simulink model "ZSM_TeslaModelS_statKreisfahrt"  (R2020b)
settings: Solver=FixedStepDiscrete  StartTime=0.0  StopTime=simtime  FixedStep=stepsize  RelTol=1e-3
undefined symbols (not defined in the file): activate_stop, activate_stop_vmax, ay_stop, ayObs, ayStiff, Bat_param, deltav_ist, DiscIntNeverNeededParam, EG_wunsch, magnitude, mu_road_LF, mu_road_LR, mu_road_RF, mu_road_RR, par_ASR, par_MDT, par_TIR, par_VEH, select_delta_h, select_M_wheel, stepsize, t, temp_betriebsstrategie, temperature_LTrange, track_left, track_right
libraries: Library_ASK x36, simulink x16, pid_lib x2, dspstat3 x2, Library_Betriebsstrategie x2, vehicle_model x2, pacejka_trans x1
(part 6 of 7)

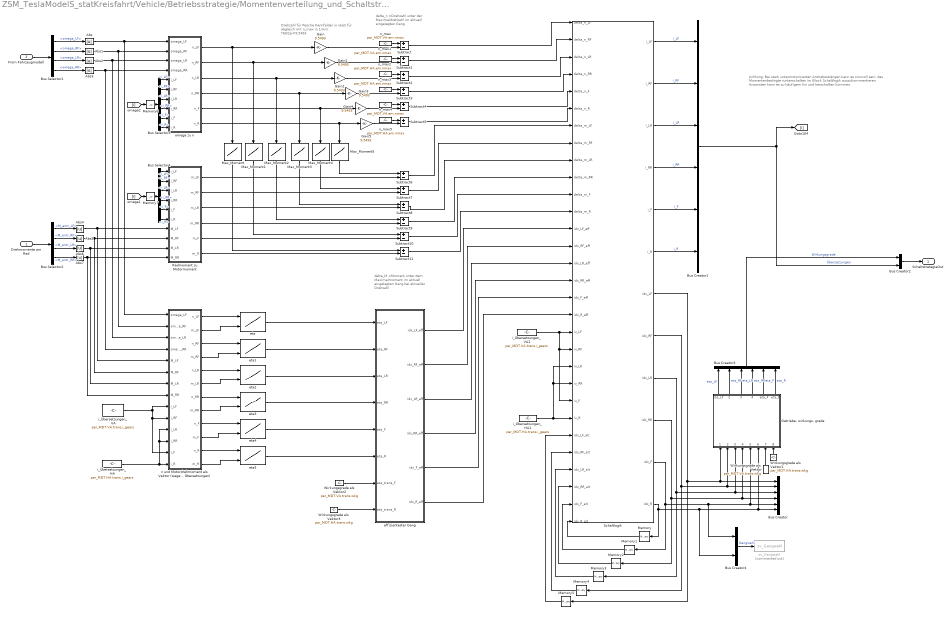
== system ZSM_TeslaModelS_statKreisfahrt/Vehicle/Betriebsstrategie/Momentenverteilung_und_Schaltstrategie1/Radmomentenaufteilung (Standardfahrmanöver)/Schaltstrategie ==
  note: Drehzahl für Pesche Kennfelder in rad/s
      | für abgleich mit n_max in 1/min
      | *60/2pi=9.5493
  note: Achtung: Bei stark untermotorisierten Antriebssträngen kann es sinnvoll sein,
      | das Momentenbedingte runterschalten im Block Schaltlogik auszukommentieren.
      | Ansonsten kann es zu häufigem hin und herschalten kommen.
  note: delta_M =Moment unter dem Maximalmoment im aktuell eingelegten Gang bei aktueller Drehzahl
  note: delta_n =Drehzahl unter der Maximaldrehzahl im aktuell eingelegten Gang
  Drehmomente am Rad : Inport
  From Fahrzeugmodell : Inport  Port=2
  Abs{,1..7} (8 alike) : Abs
  Bus Creator : BusCreator  Inputs=6
  Bus Creator1 : BusCreator  Inputs=6
  Bus Creator2 : BusCreator  Inputs=2
  Bus Creator3 : BusCreator  Inputs=6
  Bus Creator4 : BusCreator  Inputs=2
  Bus Selector1 : BusSelector  OutputSignals=omega.omega_LF,omega.omega_RF,omega.omega_LR,omega.omega_RR
  Bus Selector2 : BusSelector  OutputSignals=M_antr_LF,M_antr_RF,M_antr_LR,M_antr_RR
  Bus Selector3 : BusSelector  OutputSignals=i_LF,i_RF,i_LR,i_RR,i_F,i_R
  Bus Selector4 : BusSelector  OutputSignals=i_LF,i_RF,i_LR,i_RR,i_F,i_R
  Gain{,1..5} (6 alike) : Gain  Gain=9.5493
  Getriebe- wirkungs- grade : MATLAB Function  TreatAsAtomicUnit=on
  Max_Moment : Lookup_n-D  NumberOfTableDimensions=1  BreakpointsForDimension1=par_MDT.VA.em.MaxMotorTrqCurve_w  Table=par_MDT.VA.em.MaxMotorTrqCurve_M  InternalRulePriority=Speed  RndMeth=Simplest  InputSameDT=on
  Max_Moment1 : Lookup_n-D  NumberOfTableDimensions=1  BreakpointsForDimension1=par_MDT.VA.em.MaxMotorTrqCurve_w  Table=par_MDT.VA.em.MaxMotorTrqCurve_M  InternalRulePriority=Speed  RndMeth=Simplest  InputSameDT=on
  Max_Moment2 : Lookup_n-D  NumberOfTableDimensions=1  BreakpointsForDimension1=par_MDT.HA.em.MaxMotorTrqCurve_w  Table=par_MDT.HA.em.MaxMotorTrqCurve_M  InternalRulePriority=Speed  RndMeth=Simplest  InputSameDT=on
  Max_Moment3 : Lookup_n-D  NumberOfTableDimensions=1  BreakpointsForDimension1=par_MDT.HA.em.MaxMotorTrqCurve_w  Table=par_MDT.HA.em.MaxMotorTrqCurve_M  InternalRulePriority=Speed  RndMeth=Simplest  InputSameDT=on
  Max_Moment4 : Lookup_n-D  NumberOfTableDimensions=1  BreakpointsForDimension1=par_MDT.VA.em.MaxMotorTrqCurve_w  Table=par_MDT.VA.em.MaxMotorTrqCurve_M  InternalRulePriority=Speed  RndMeth=Simplest  InputSameDT=on
  Max_Moment5 : Lookup_n-D  NumberOfTableDimensions=1  BreakpointsForDimension1=par_MDT.HA.em.MaxMotorTrqCurve_w  Table=par_MDT.HA.em.MaxMotorTrqCurve_M  InternalRulePriority=Speed  RndMeth=Simplest  InputSameDT=on
  Memory{,1..7} (8 alike) : Memory  InitialCondition=1
  Radmoment zu Motormoment : MATLAB Function  TreatAsAtomicUnit=on
  Schaltlogik : MATLAB Function  TreatAsAtomicUnit=on
  Subtract{,1..11} (12 alike) : Sum  Inputs=+-
  Wirkungsgrade als Vektor : Constant  Value=par_MDT.VA.trans.wkg
  Wirkungsgrade als Vektor1 : Constant  Value=par_MDT.HA.trans.wkg
  Wirkungsgrade als Vektor2 : Constant  Value=par_MDT.VA.trans.wkg
  Wirkungsgrade als Vektor3 : Constant  Value=par_MDT.HA.trans.wkg
  effizientester Gang : MATLAB Function  TreatAsAtomicUnit=on
  eta : Lookup_n-D  BreakpointsForDimension1=par_MDT.VA.em.MotorEffMap3D_w  BreakpointsForDimension2=par_MDT.VA.em.MotorEffMap3D_M  Table=par_MDT.VA.em.MotorEffMap3D  InternalRulePriority=Speed  RndMeth=Simplest  InputSameDT=on
      settings: InputPortMap=u0,u1
  eta1 : Lookup_n-D  BreakpointsForDimension1=par_MDT.VA.em.MotorEffMap3D_w  BreakpointsForDimension2=par_MDT.VA.em.MotorEffMap3D_M  Table=par_MDT.VA.em.MotorEffMap3D  InternalRulePriority=Speed  RndMeth=Simplest  InputSameDT=on
      settings: InputPortMap=u0,u1
  eta2 : Lookup_n-D  BreakpointsForDimension1=par_MDT.HA.em.MotorEffMap3D_w  BreakpointsForDimension2=par_MDT.HA.em.MotorEffMap3D_M  Table=par_MDT.HA.em.MotorEffMap3D  InternalRulePriority=Speed  RndMeth=Simplest  InputSameDT=on
      settings: InputPortMap=u0,u1
  eta3 : Lookup_n-D  BreakpointsForDimension1=par_MDT.HA.em.MotorEffMap3D_w  BreakpointsForDimension2=par_MDT.HA.em.MotorEffMap3D_M  Table=par_MDT.HA.em.MotorEffMap3D  InternalRulePriority=Speed  RndMeth=Simplest  InputSameDT=on
      settings: InputPortMap=u0,u1
  eta4 : Lookup_n-D  BreakpointsForDimension1=par_MDT.VA.em.MotorEffMap3D_w  BreakpointsForDimension2=par_MDT.VA.em.MotorEffMap3D_M  Table=par_MDT.VA.em.MotorEffMap3D  InternalRulePriority=Speed  RndMeth=Simplest  InputSameDT=on
      settings: InputPortMap=u0,u1
  eta5 : Lookup_n-D  BreakpointsForDimension1=par_MDT.HA.em.MotorEffMap3D_w  BreakpointsForDimension2=par_MDT.HA.em.MotorEffMap3D_M  Table=par_MDT.HA.em.MotorEffMap3D  InternalRulePriority=Speed  RndMeth=Simplest  InputSameDT=on
      settings: InputPortMap=u0,u1
  i_Übersetzungen_HA : Constant  Value=par_MDT.HA.trans.i_gears
  i_Übersetzungen_HA1 : Constant  Value=par_MDT.HA.trans.i_gears
  i_Übersetzungen_VA : Constant  Value=par_MDT.VA.trans.i_gears
  i_Übersetzungen_VA1 : Constant  Value=par_MDT.VA.trans.i_gears
  n und Motordrehmoment als Vektor (wegen ALLEN Übersetzungen) : MATLAB Function  TreatAsAtomicUnit=on
  n_max : Constant  Value=par_MDT.VA.em.nmax
  n_max1 : Constant  Value=par_MDT.VA.em.nmax
  n_max2 : Constant  Value=par_MDT.HA.em.nmax
  n_max3 : Constant  Value=par_MDT.HA.em.nmax
  n_max4 : Constant  Value=par_MDT.VA.em.nmax
  n_max5 : Constant  Value=par_MDT.HA.em.nmax
  omega zu n : MATLAB Function  TreatAsAtomicUnit=on
  sv_Gangwahl : ToWorkspace  Commented=on  VariableName=sv_Gangwahl  SaveFormat=Timeseries  SampleTime=-1
      settings: Decimation=savedec
  SchaltstrategieOut : Outport  VectorParamsAs1DForOutWhenUnconnected=off
  wires:
  Abs7/1 -> n und Motordrehmoment als Vektor (wegen ALLEN Übersetzungen)/8(M_RR), Radmoment zu Motormoment/10(M_RR)
  Abs6/1 -> n und Motordrehmoment als Vektor (wegen ALLEN Übersetzungen)/7(M_LR), Radmoment zu Motormoment/9(M_LR)
  Abs5/1 -> n und Motordrehmoment als Vektor (wegen ALLEN Übersetzungen)/6(M_RF), Radmoment zu Motormoment/8(M_RF)
  Abs4/1 -> n und Motordrehmoment als Vektor (wegen ALLEN Übersetzungen)/5(M_LF), Radmoment zu Motormoment/7(M_LF)
  Abs3/1 -> n und Motordrehmoment als Vektor (wegen ALLEN Übersetzungen)/4(omega_RR), omega zu n/4(omega_RR)
  Abs2/1 -> n und Motordrehmoment als Vektor (wegen ALLEN Übersetzungen)/3(omega_LR), omega zu n/3(omega_LR)
  Abs1/1 -> n und Motordrehmoment als Vektor (wegen ALLEN Übersetzungen)/2(omega_RF), omega zu n/2(omega_RF)
  Abs/1 -> n und Motordrehmoment als Vektor (wegen ALLEN Übersetzungen)/1(omega_LF), omega zu n/1(omega_LF)
  omega zu n/6(n_R) -> Gain5/1, Max_Moment5/1
  omega zu n/1(n_LF) -> Gain/1, Max_Moment/1
  omega zu n/5(n_F) -> Max_Moment4/1, Gain4/1
  omega zu n/4(n_RR) -> Max_Moment3/1, Gain3/1
  omega zu n/3(n_LR) -> Max_Moment2/1, Gain2/1
  omega zu n/2(n_RF) -> Max_Moment1/1, Gain1/1
  Bus Selector1/4 -> Abs3/1  "<omega_RR>"
  Bus Selector1/3 -> Abs2/1  "<omega_LR>"
  Bus Selector1/2 -> Abs1/1  "<omega_RF>"
  Bus Selector1/1 -> Abs/1  "<omega_LF>"
  Drehmomente am Rad/1 -> Bus Selector2/1
  From Fahrzeugmodell/1 -> Bus Selector1/1
  Bus Selector2/1 -> Abs4/1  "<M_antr_LF>"
  Bus Selector2/2 -> Abs5/1  "<M_antr_RF>"
  Bus Selector2/3 -> Abs6/1  "<M_antr_LR>"
  Bus Selector2/4 -> Abs7/1  "<M_antr_RR>"
  n_max/1 -> Subtract/1
  n_max1/1 -> Subtract1/1
  n_max2/1 -> Subtract2/1
  n_max3/1 -> Subtract3/1
  n_max4/1 -> Subtract4/1
  n_max5/1 -> Subtract5/1
  Radmoment zu Motormoment/1(m_LF) -> Subtract6/2
  Radmoment zu Motormoment/2(m_RF) -> Subtract7/2
  Radmoment zu Motormoment/3(m_LR) -> Subtract8/2
  Radmoment zu Motormoment/4(m_RR) -> Subtract9/2
  Radmoment zu Motormoment/5(m_F) -> Subtract10/2
  Radmoment zu Motormoment/6(m_R) -> Subtract11/2
  Max_Moment5/1 -> Subtract6/1
  Max_Moment4/1 -> Subtract7/1
  Max_Moment3/1 -> Subtract8/1
  Max_Moment2/1 -> Subtract9/1
  Max_Moment1/1 -> Subtract10/1
  Max_Moment/1 -> Subtract11/1
  i_Übersetzungen_VA/1 -> n und Motordrehmoment als Vektor (wegen ALLEN Übersetzungen)/9(i_LF), n und Motordrehmoment als Vektor (wegen ALLEN Übersetzungen)/13(i_F), n und Motordrehmoment als Vektor (wegen ALLEN Übersetzungen)/10(i_RF)
  n und Motordrehmoment als Vektor (wegen ALLEN Übersetzungen)/1(n_LF) -> eta/1
  n und Motordrehmoment als Vektor (wegen ALLEN Übersetzungen)/2(m_LF) -> eta/2
  n und Motordrehmoment als Vektor (wegen ALLEN Übersetzungen)/3(n_RF) -> eta1/1
  n und Motordrehmoment als Vektor (wegen ALLEN Übersetzungen)/4(m_RF) -> eta1/2
  n und Motordrehmoment als Vektor (wegen ALLEN Übersetzungen)/5(n_LR) -> eta2/1
  n und Motordrehmoment als Vektor (wegen ALLEN Übersetzungen)/6(m_LR) -> eta2/2
  n und Motordrehmoment als Vektor (wegen ALLEN Übersetzungen)/7(n_RR) -> eta3/1
  n und Motordrehmoment als Vektor (wegen ALLEN Übersetzungen)/8(m_RR) -> eta3/2
  n und Motordrehmoment als Vektor (wegen ALLEN Übersetzungen)/9(n_F) -> eta4/1
  n und Motordrehmoment als Vektor (wegen ALLEN Übersetzungen)/10(m_F) -> eta4/2
  n und Motordrehmoment als Vektor (wegen ALLEN Übersetzungen)/11(n_R) -> eta5/1
  n und Motordrehmoment als Vektor (wegen ALLEN Übersetzungen)/12(m_R) -> eta5/2
  eta/1 -> effizientester Gang/1(eta_LF)
  eta1/1 -> effizientester Gang/2(eta_RF)
  eta2/1 -> effizientester Gang/3(eta_LR)
  eta3/1 -> effizientester Gang/4(eta_RR)
  eta4/1 -> effizientester Gang/5(eta_F)
  eta5/1 -> effizientester Gang/6(eta_R)
  Subtract/1 -> Schaltlogik/1(delta_n_LF)
  Subtract1/1 -> Schaltlogik/2(delta_n_RF)
  Subtract2/1 -> Schaltlogik/3(delta_n_LR)
  Subtract3/1 -> Schaltlogik/4(delta_n_RR)
  Subtract4/1 -> Schaltlogik/5(delta_n_F)
  Subtract5/1 -> Schaltlogik/6(delta_n_R)
  Subtract6/1 -> Schaltlogik/7(delta_m_LF)
  Subtract7/1 -> Schaltlogik/8(delta_m_RF)
  Subtract8/1 -> Schaltlogik/9(delta_m_LR)
  Subtract9/1 -> Schaltlogik/10(delta_m_RR)
  Subtract10/1 -> Schaltlogik/11(delta_m_F)
  Subtract11/1 -> Schaltlogik/12(delta_m_R)
  effizientester Gang/1(idx_LF_eff) -> Schaltlogik/13(idx_LF_eff)
  effizientester Gang/2(idx_RF_eff) -> Schaltlogik/14(idx_RF_eff)
  effizientester Gang/3(idx_LR_eff) -> Schaltlogik/15(idx_LR_eff)
  effizientester Gang/4(idx_RR_eff) -> Schaltlogik/16(idx_RR_eff)
  effizientester Gang/5(idx_F_eff) -> Schaltlogik/17(idx_F_eff)
  effizientester Gang/6(idx_R_eff) -> Schaltlogik/18(idx_R_eff)
  Schaltlogik/12(idx_R) -> Memory/1, Bus Creator4/2, Getriebe- wirkungs- grade/6(idx_R), Bus Creator/6
  Schaltlogik/11(idx_F) -> Memory1/1, Bus Creator4/1, Bus Creator/5, Getriebe- wirkungs- grade/5(idx_F)
  Schaltlogik/9(idx_LR) -> Memory3/1, Bus Creator/3, Getriebe- wirkungs- grade/3(idx_LR)
  Schaltlogik/8(idx_RF) -> Memory4/1, Bus Creator/2, Getriebe- wirkungs- grade/2(idx_RF)
  Schaltlogik/7(idx_LF) -> Memory5/1, Bus Creator/1, Getriebe- wirkungs- grade/1(idx_LF)
  Memory/1 -> Schaltlogik/30(idx_R_alt)
  Memory1/1 -> Schaltlogik/29(idx_F_alt)
  Memory2/1 -> Schaltlogik/28(idx_RR_alt)
  Memory3/1 -> Schaltlogik/27(idx_LR_alt)
  Memory4/1 -> Schaltlogik/26(idx_RF_alt)
  Memory5/1 -> Schaltlogik/25(idx_LF_alt)
  Schaltlogik/10(idx_RR) -> Memory2/1, Bus Creator/4, Getriebe- wirkungs- grade/4(idx_RR)
  Schaltlogik/1(i_LF) -> Bus Creator1/1  "i_LF"
  Schaltlogik/2(i_RF) -> Bus Creator1/2  "i_RF"
  Schaltlogik/3(i_LR) -> Bus Creator1/3  "i_LR"
  Schaltlogik/4(i_RR) -> Bus Creator1/4  "i_RR"
  Schaltlogik/5(i_F) -> Bus Creator1/5  "i_F"
  Schaltlogik/6(i_R) -> Bus Creator1/6  "i_R"
  Bus Selector3/1 -> omega zu n/5(i_LF)  "<i_LF>"
  [i] -> Memory6/1
  Bus Selector3/2 -> omega zu n/6(i_RF)  "<i_RF>"
  Bus Selector3/3 -> omega zu n/7(i_LR)  "<i_LR>"
  Bus Selector3/4 -> omega zu n/8(i_RR)  "<i_RR>"
  Bus Selector3/5 -> omega zu n/9(i_F)  "<i_F>"
  Bus Selector3/6 -> omega zu n/10(i_R)  "<i_R>"
  Memory6/1 -> Bus Selector3/1
  [i] -> Memory7/1
  Memory7/1 -> Bus Selector4/1
  Bus Selector4/1 -> Radmoment zu Motormoment/1(i_LF)  "<i_LF>"
  Bus Selector4/2 -> Radmoment zu Motormoment/2(i_RF)  "<i_RF>"
  Bus Selector4/3 -> Radmoment zu Motormoment/3(i_LR)  "<i_LR>"
  Bus Selector4/4 -> Radmoment zu Motormoment/4(i_RR)  "<i_RR>"
  Bus Selector4/5 -> Radmoment zu Motormoment/5(i_F)  "<i_F>"
  Bus Selector4/6 -> Radmoment zu Motormoment/6(i_R)  "<i_R>"
  i_Übersetzungen_HA/1 -> n und Motordrehmoment als Vektor (wegen ALLEN Übersetzungen)/11(i_LR), n und Motordrehmoment als Vektor (wegen ALLEN Übersetzungen)/12(i_RR), n und Motordrehmoment als Vektor (wegen ALLEN Übersetzungen)/14(i_R)
  i_Übersetzungen_VA1/1 -> Schaltlogik/23(iv_F), Schaltlogik/20(iv_RF), Schaltlogik/19(iv_LF)
  i_Übersetzungen_HA1/1 -> Schaltlogik/21(iv_LR), Schaltlogik/22(iv_RR), Schaltlogik/24(iv_R)
  Gain/1 -> Subtract/2
  Gain1/1 -> Subtract1/2
  Gain2/1 -> Subtract2/2
  Gain3/1 -> Subtract3/2
  Gain4/1 -> Subtract4/2
  Gain5/1 -> Subtract5/2
  Bus Creator1/1 -> Bus Creator2/2, [i]  "Übersetzungen"
  Bus Creator2/1 -> SchaltstrategieOut/1
  Wirkungsgrade als Vektor/1 -> Getriebe- wirkungs- grade/7(ETA_F)
  Wirkungsgrade als Vektor1/1 -> Getriebe- wirkungs- grade/8(ETA_R)
  Getriebe- wirkungs- grade/2(eta_RF) -> Bus Creator3/2  "eta_RF"
  Getriebe- wirkungs- grade/3(eta_LR) -> Bus Creator3/3  "eta_LR"
  Getriebe- wirkungs- grade/4(eta_RR) -> Bus Creator3/4  "eta_RR"
  Getriebe- wirkungs- grade/5(eta_F) -> Bus Creator3/5  "eta_F"
  Getriebe- wirkungs- grade/6(eta_R) -> Bus Creator3/6  "eta_R"
  Getriebe- wirkungs- grade/1(eta_LF) -> Bus Creator3/1  "eta_LF"
  Bus Creator3/1 -> Bus Creator2/1  "Wirkungsgrade"
  Wirkungsgrade als Vektor2/1 -> effizientester Gang/7(eta_trans_F)
  Wirkungsgrade als Vektor3/1 -> effizientester Gang/8(eta_trans_R)
  Bus Creator4/1 -> sv_Gangwahl/1  "Gangwahl"

== system ZSM_TeslaModelS_statKreisfahrt/Vehicle/Betriebsstrategie/Momentenverteilung_und_Schaltstrategie1/adaptive Limiter/Enabled Subsystem ==
  In1 : Inport
  Enable : EnablePort
  Out1 : Outport  VectorParamsAs1DForOutWhenUnconnected=off
  wires:
  In1/1 -> Out1/1

== system ZSM_TeslaModelS_statKreisfahrt/Vehicle/Betriebsstrategie/Momentenverteilung_und_Schaltstrategie1/adaptive Limiter/Enabled Subsystem1 ==
  In1 : Inport
  Enable : EnablePort
  Discrete-Time Integrator : DiscreteIntegrator  InitialCondition=1  SampleTime=-1  ICPrevOutput=DiscIntNeverNeededParam  ICPrevScaledInput=DiscIntNeverNeededParam
  Out1 : Outport  VectorParamsAs1DForOutWhenUnconnected=off
  wires:
  Discrete-Time Integrator/1 -> Out1/1
  In1/1 -> Discrete-Time Integrator/1

== system ZSM_TeslaModelS_statKreisfahrt/Vehicle/Betriebsstrategie/Momentenverteilung_und_Schaltstrategie1/Radmomentenaufteilung (Effizienz)/Limits ermitteln/Axle activator ==
  Add4 : Sum
  Add6 : Sum
  Constant3 : Constant  Value=par_MDT.AUS.akt.az_VA
  Constant4 : Constant  Value=par_MDT.AUS.akt.az_HA
  Constant5 : Constant  Value=par_MDT.AUS.akt.rn_HA
  Constant6 : Constant  Value=par_MDT.AUS.akt.rn_VA
  VA : Outport  VectorParamsAs1DForOutWhenUnconnected=off
  HA : Outport  Port=2  VectorParamsAs1DForOutWhenUnconnected=off
  wires:
  Add4/1 -> VA/1
  Constant6/1 -> Add4/2
  Constant3/1 -> Add4/1
  Constant5/1 -> Add6/2
  Add6/1 -> HA/1
  Constant4/1 -> Add6/1

== system ZSM_TeslaModelS_statKreisfahrt/Vehicle/Betriebsstrategie/Momentenverteilung_und_Schaltstrategie1/Radmomentenaufteilung (Effizienz)/Limits ermitteln/Falls M_wheel kleiner als M_VA_pot ==
  M_VA_pot_in : Inport
  M_wheel : Inport  Port=2
  Rekuindex : Inport  Port=3
  M_HA_pot_in : Inport  Port=4
  Abs : Abs
  Abs1 : Abs
  Abs2 : Abs
  MinMax : MinMax  Inputs=2
  MinMax1 : MinMax  Inputs=2
  Product : Product
  Product1 : Product
  M_VA_pot_out : Outport  VectorParamsAs1DForOutWhenUnconnected=off
  M_wheel_out : Outport  Port=2  VectorParamsAs1DForOutWhenUnconnected=off
  M_HA_pot_out : Outport  Port=3  VectorParamsAs1DForOutWhenUnconnected=off
  wires:
  Abs1/1 -> MinMax1/1, MinMax/2
  MinMax/1 -> Product/1
  Abs/1 -> MinMax/1
  M_VA_pot_in/1 -> Abs/1
  M_wheel/1 -> M_wheel_out/1, Abs1/1
  Rekuindex/1 -> Product1/1, Product/2
  Product/1 -> M_VA_pot_out/1
  Abs2/1 -> MinMax1/2
  M_HA_pot_in/1 -> Abs2/1
  MinMax1/1 -> Product1/2
  Product1/1 -> M_HA_pot_out/1

== system ZSM_TeslaModelS_statKreisfahrt/Vehicle/Betriebsstrategie/Momentenverteilung_und_Schaltstrategie1/Radmomentenaufteilung (Effizienz)/Momentenrückführung und Motormomentberechnung/Getriebewirkungsgradberechnung Hinterachse ==
  Rekuindex : Inport
  M_HA_mot : Inport  Port=2
  Abs : Abs
  Constant1 : Constant  Value=par_VEH.dt.ecu.Wirkungsgrade_HA
  Constant2 : Constant  Commented=on  Value=par_MDT.HA.em.M_max_achse
  Divide : Product  Commented=on  Inputs=*/
  Divide1 : Product  Inputs=/*
  Falls radnahe Maschine an HA1 : Subsystem
  Falls radnahe Maschine an HA2 : Subsystem
  MATLAB Function1 : MATLAB Function  Commented=on  TreatAsAtomicUnit=on
  Product : Product
  Switch : Switch  Commented=on  Criteria=u2 > Threshold  Threshold=0.15
  WKG_GTR_HA : Outport  VectorParamsAs1DForOutWhenUnconnected=off
  wires:
  Constant2/1 -> Divide/2, MATLAB Function1/2(M_max)
  Constant1/1 -> Divide1/1
  M_HA_mot/1 -> Abs/1
  Product/1 -> Falls radnahe Maschine an HA2/1(M_HA)
  Falls radnahe Maschine an HA1/1(M_HA_mot) -> Divide1/2
  ? -> Switch/1, Divide/1, MATLAB Function1/1(M_out)
  Switch/1 -> ?
  Rekuindex/1 -> Product/2
  Abs/1 -> Falls radnahe Maschine an HA1/1(M_HA)
  MATLAB Function1/1(M_in) -> Switch/3
  Divide/1 -> Switch/2
  Falls radnahe Maschine an HA2/1(M_HA_mot) -> WKG_GTR_HA/1
  Divide1/1 -> Product/1

== system ZSM_TeslaModelS_statKreisfahrt/Vehicle/Betriebsstrategie/Momentenverteilung_und_Schaltstrategie1/Radmomentenaufteilung (Effizienz)/Momentenrückführung und Motormomentberechnung/Getriebewirkungsgradberechnung Vorderachse ==
  M_VA_mot : Inport
  Rekuindex : Inport  Port=2
  Abs : Abs
  Constant5 : Constant  Value=par_VEH.dt.ecu.Wirkungsgrade_VA
  Constant6 : Constant  Commented=on  Value=par_MDT.VA.em.M_max_achse
  Divide : Product  Commented=on  Inputs=*/
  Divide4 : Product  Inputs=/*
  Falls radnahe Maschine an VA : Subsystem
  Falls radnahe Maschine an VA1 : Subsystem
  MATLAB Function : MATLAB Function  Commented=on  TreatAsAtomicUnit=on
  Product : Product
  Switch : Switch  Commented=on  Criteria=u2 > Threshold  Threshold=0.15
  WKG_GTR_VA : Outport  VectorParamsAs1DForOutWhenUnconnected=off
  wires:
  Constant6/1 -> Divide/2, MATLAB Function/2(M_max)
  Constant5/1 -> Divide4/1
  M_VA_mot/1 -> Abs/1
  Product/1 -> Falls radnahe Maschine an VA1/1(M_VA)
  Falls radnahe Maschine an VA/1(M_VA_mot) -> Divide4/2
  ? -> Switch/1, Divide/1, MATLAB Function/1(M_out)
  Switch/1 -> ?
  Rekuindex/1 -> Product/2
  Abs/1 -> Falls radnahe Maschine an VA/1(M_VA)
  MATLAB Function/1(M_in) -> Switch/3
  Divide/1 -> Switch/2
  Falls radnahe Maschine an VA1/1(M_VA_mot) -> WKG_GTR_VA/1
  Divide4/1 -> Product/1

== system ZSM_TeslaModelS_statKreisfahrt/Vehicle/Betriebsstrategie/Momentenverteilung_und_Schaltstrategie1/Radmomentenaufteilung (Effizienz)/Momentenrückführung und Motormomentberechnung/Subsystem ==
  M_VA_pot : Inport
  M_VA_mot_in : Inport  Port=2
  Enable : EnablePort
  Abs : Abs
  Abs1 : Abs
  Bias : Bias  Bias=0.01
  Constant1 : Constant  Value=par_VEH.dt.ecu.Wirkungsgrade_VA
  Constant4 : Constant  Value=NaN
  Divide : Product  Inputs=/*
  Relational Operator : RelationalOperator  Operator=<  OutDataTypeStr=boolean  RndMeth=Nearest
  Switch : Switch  Criteria=u2 > Threshold
  M_VA_mot_out : Outport  VectorParamsAs1DForOutWhenUnconnected=off
  wires:
  Abs/1 -> Relational Operator/2
  Switch/1 -> M_VA_mot_out/1
  Constant1/1 -> Divide/1
  M_VA_pot/1 -> Divide/2
  Bias/1 -> Relational Operator/1
  Relational Operator/1 -> Switch/2
  Constant4/1 -> Switch/1
  Divide/1 -> Abs1/1
  Abs1/1 -> Bias/1
  M_VA_mot_in/1 -> Switch/3, Abs/1

== system ZSM_TeslaModelS_statKreisfahrt/Vehicle/Betriebsstrategie/Momentenverteilung_und_Schaltstrategie1/Radmomentenaufteilung (Effizienz)/Momentenrückführung und Motormomentberechnung/Subsystem1 ==
  M_HA_pot : Inport
  M_HA_mot_in : Inport  Port=2
  Enable : EnablePort
  Abs : Abs
  Abs1 : Abs
  Bias : Bias  Bias=0.01
  Constant1 : Constant  Value=par_VEH.dt.ecu.Wirkungsgrade_HA
  Constant4 : Constant  Value=NaN
  Divide : Product  Inputs=/*
  Relational Operator : RelationalOperator  Operator=<  OutDataTypeStr=boolean  RndMeth=Nearest
  Switch : Switch  Criteria=u2 > Threshold
  M_HA_mot_out : Outport  VectorParamsAs1DForOutWhenUnconnected=off
  wires:
  Abs1/1 -> Bias/1
  Abs/1 -> Relational Operator/2
  Switch/1 -> M_HA_mot_out/1
  Bias/1 -> Relational Operator/1
  M_HA_mot_in/1 -> Switch/3, Abs/1
  Constant4/1 -> Switch/1
  Relational Operator/1 -> Switch/2
  Divide/1 -> Abs1/1
  M_HA_pot/1 -> Divide/2
  Constant1/1 -> Divide/1

== system ZSM_TeslaModelS_statKreisfahrt/Vehicle/Betriebsstrategie/Momentenverteilung_und_Schaltstrategie1/Radmomentenaufteilung (Effizienz)/Optimierung und Schaltstrategie/Bereinigung ==
  M_VA_in : Inport
  M_HA_in : Inport  Port=2
  Constant : Constant  Value=0
  Constant1 : Constant  Value=0
  Relational Operator : RelationalOperator  Operator=isNaN  OutDataTypeStr=boolean  RndMeth=Nearest
  Relational Operator1 : RelationalOperator  Operator=isNaN  OutDataTypeStr=boolean  RndMeth=Nearest
  Switch : Switch  Criteria=u2 > Threshold
  Switch1 : Switch  Criteria=u2 > Threshold
  M_VA_out : Outport  VectorParamsAs1DForOutWhenUnconnected=off
  M_HA_out : Outport  Port=2  VectorParamsAs1DForOutWhenUnconnected=off
  wires:
  Switch1/1 -> M_HA_out/1
  M_VA_in/1 -> Relational Operator/1, Switch/3
  Constant/1 -> Switch/1
  Switch/1 -> M_VA_out/1
  Constant1/1 -> Switch1/1
  Relational Operator1/1 -> Switch1/2
  M_HA_in/1 -> Relational Operator1/1, Switch1/3
  Relational Operator/1 -> Switch/2

== system ZSM_TeslaModelS_statKreisfahrt/Vehicle/Betriebsstrategie/Momentenverteilung_und_Schaltstrategie1/Radmomentenaufteilung (Effizienz)/Torque shift damper/Axle activator ==
  Add4 : Sum
  Add6 : Sum
  Constant3 : Constant  Value=par_MDT.AUS.akt.az_VA
  Constant4 : Constant  Value=par_MDT.AUS.akt.az_HA
  Constant5 : Constant  Value=par_MDT.AUS.akt.rn_HA
  Constant6 : Constant  Value=par_MDT.AUS.akt.rn_VA
  VA : Outport  VectorParamsAs1DForOutWhenUnconnected=off
  HA : Outport  Port=2  VectorParamsAs1DForOutWhenUnconnected=off
  wires:
  Add4/1 -> VA/1
  Constant6/1 -> Add4/2
  Constant3/1 -> Add4/1
  Constant5/1 -> Add6/2
  Add6/1 -> HA/1
  Constant4/1 -> Add6/1

== system ZSM_TeslaModelS_statKreisfahrt/Vehicle/Betriebsstrategie/Momentenverteilung_und_Schaltstrategie1/Radmomentenaufteilung (Effizienz)/Torque shift damper/Optimierung_damped_AWD ==
  P_achs : Inport
  M_target : Inport  Port=2
  Enable : EnablePort
  Constant : Constant  Value=0.022
  Constant1 : Constant  Value=2
  Memory : Memory  InitialCondition=1
  Memory1 : Memory
  Memory2 : Memory  InitialCondition=1
  Minimierung : MATLAB Function  TreatAsAtomicUnit=on
  Product : Product
  Sign : Signum
  P_opt : Outport  VectorParamsAs1DForOutWhenUnconnected=off
  ind : Outport  Port=2  VectorParamsAs1DForOutWhenUnconnected=off
  wires:
  P_achs/1 -> Minimierung/1(P_achs)
  M_target/1 -> Product/1, Minimierung/4(M_target), Memory2/1
  Constant/1 -> Minimierung/2(difference)
  Memory2/1 -> Product/2
  Constant1/1 -> Minimierung/3(max_oscillation_sec)
  Minimierung/2(ind) -> ind/1, Memory/1
  Memory1/1 -> Minimierung/7(count_prev)
  Memory/1 -> Minimierung/6(ind_prev)
  Minimierung/3(count) -> Memory1/1
  Minimierung/1(P_opt) -> P_opt/1
  Product/1 -> Sign/1
  Sign/1 -> Minimierung/5(change)

== system ZSM_TeslaModelS_statKreisfahrt/Vehicle/Betriebsstrategie/Momentenverteilung_und_Schaltstrategie1/Radmomentenaufteilung (Effizienz)/Torque shift damper/Optimierung_eine_achs ==
  P_achs : Inport
  M_target : Inport  Port=2
  Akt_VA : Inport  Port=3
  Akt_HA : Inport  Port=4
  Enable : EnablePort
  Optimierung : MATLAB Function  TreatAsAtomicUnit=on
  "P_opt " : Outport  VectorParamsAs1DForOutWhenUnconnected=off
  "ind " : Outport  Port=2  VectorParamsAs1DForOutWhenUnconnected=off
  wires:
  Optimierung/1(P_opt) -> "P_opt "/1
  Optimierung/2(ind) -> "ind "/1
  M_target/1 -> Optimierung/2(M_target)
  P_achs/1 -> Optimierung/1(P_achs)
  Akt_VA/1 -> Optimierung/3(VA)
  Akt_HA/1 -> Optimierung/4(HA)

== system ZSM_TeslaModelS_statKreisfahrt/Vehicle/Betriebsstrategie/Momentenverteilung_und_Schaltstrategie1/Radmomentenaufteilung (Effizienz)/Momentenrückführung und Motormomentberechnung/Getriebewirkungsgradberechnung Hinterachse/Falls radnahe Maschine an HA1 ==
  M_HA : Inport
  Constant1 : Constant  Value=par_MDT.AUS.akt.az_HA
  Gain : Gain  Gain=0.5
  Switch : Switch  Criteria=u2 > Threshold
  M_HA_mot : Outport  VectorParamsAs1DForOutWhenUnconnected=off
  wires:
  Constant1/1 -> Switch/2
  M_HA/1 -> Switch/1, Gain/1
  Gain/1 -> Switch/3
  Switch/1 -> M_HA_mot/1

== system ZSM_TeslaModelS_statKreisfahrt/Vehicle/Betriebsstrategie/Momentenverteilung_und_Schaltstrategie1/Radmomentenaufteilung (Effizienz)/Momentenrückführung und Motormomentberechnung/Getriebewirkungsgradberechnung Hinterachse/Falls radnahe Maschine an HA2 ==
  M_HA : Inport
  Constant1 : Constant  Value=par_MDT.AUS.akt.az_HA
  Gain : Gain  Gain=2
  Switch : Switch  Criteria=u2 > Threshold
  M_HA_mot : Outport  VectorParamsAs1DForOutWhenUnconnected=off
  wires:
  Constant1/1 -> Switch/2
  M_HA/1 -> Switch/1, Gain/1
  Gain/1 -> Switch/3
  Switch/1 -> M_HA_mot/1

== system ZSM_TeslaModelS_statKreisfahrt/Vehicle/Betriebsstrategie/Momentenverteilung_und_Schaltstrategie1/Radmomentenaufteilung (Effizienz)/Momentenrückführung und Motormomentberechnung/Getriebewirkungsgradberechnung Vorderachse/Falls radnahe Maschine an VA ==
  M_VA : Inport
  Constant1 : Constant  Value=par_MDT.AUS.akt.az_VA
  Gain : Gain  Gain=0.5
  Switch : Switch  Criteria=u2 > Threshold
  M_VA_mot : Outport  VectorParamsAs1DForOutWhenUnconnected=off
  wires:
  Constant1/1 -> Switch/2
  M_VA/1 -> Switch/1, Gain/1
  Gain/1 -> Switch/3
  Switch/1 -> M_VA_mot/1

== system ZSM_TeslaModelS_statKreisfahrt/Vehicle/Betriebsstrategie/Momentenverteilung_und_Schaltstrategie1/Radmomentenaufteilung (Effizienz)/Momentenrückführung und Motormomentberechnung/Getriebewirkungsgradberechnung Vorderachse/Falls radnahe Maschine an VA1 ==
  M_VA : Inport
  Constant1 : Constant  Value=par_MDT.AUS.akt.az_VA
  Gain : Gain  Gain=2
  Switch : Switch  Criteria=u2 > Threshold
  M_VA_mot : Outport  VectorParamsAs1DForOutWhenUnconnected=off
  wires:
  Constant1/1 -> Switch/2
  M_VA/1 -> Switch/1, Gain/1
  Gain/1 -> Switch/3
  Switch/1 -> M_VA_mot/1

== matlab function ZSM_TeslaModelS_statKreisfahrt/Driver/driver lateral/Pure Pursuit/MATLAB Function ==
  data: oldtime input; lad input; time input; v2 input; v1 input; v0 input; p3 input; p2 input; p1 input; p0 input; p_ist input; time_out output; dt output; err output; cp output
function [time_out, dt, err, cp]    = Carott(oldtime, lad, time,v2, v1, v0, p3, p2, p1, p0, p_ist)

t = oldtime; %Übernahme der Zeit aus letztem Zeitschritt

%Verhindert einen Zeitindex außerhalb der Matrixgröße
if oldtime > length(p0)-2
    oldtime = length(p0)-2;
elseif oldtime < 0
    oldtime = 0
end


si = int16(floor(oldtime)+1); %Spline Index, Auswahl des Richtigen Splines 
ov = t-floor(oldtime); %Overshoot, Zeit nach dem Beginn des Spline
cp =  p3(:,si).*(ov).^3+p2(:,si).*(ov).^2+p1(:,si).*(ov)+p0(:,si); %Berechnung des CP bei prognostizierter Zeit 


dist = norm(cp-p_ist); %Abstand Carrot-Point zum Fahrzeug
err = abs(1-dist/lad) %Normierung des Fehlers auf LAD
dt = 0; %Zeitdifferenz wird genullt

    v =  norm(v2(:,si).*(ov).^2+v1(:,si).*(ov)  +v0(:,si)); %FZG-Geschwindigkeit wird berechnet
    if v < 0.3 %Mindestgeschwindigkeit um CP bei Stillstand zu ermitteln 
        v = 0.3
    end
    dt = dt + (lad-dist)/v*100; %Zeitdifferenz wird aus Abstandsfehler und Geschwindigkeit ermittelt
    newtime = oldtime + dt; %Neuer Zeitpunkt, auf dem sich CP befindet, wird prognostiziert
    t = newtime; %Übernahme der prognostizierten Zeit
    
    %Verhindert einen Zeitindex außerhalb der Matrixgröße
    if newtime > length(p0)-2
        newtime = length(p0)-2;
    elseif newtime < 0
        newtime = 0
    end
    
    si = int16(floor(newtime)+1); %Spline Index, Auswahl des Richtigen Splines 
    ov = t-floor(newtime); %Overshoot, Zeit nach dem Beginn des Spline
    cp =  p3(:,si).*(ov).^3+p2(:,si).*(ov).^2+p1(:,si).*(ov)+p0(:,si); %Berechnung des CP bei neuer prognostizierter Zeit 
    dist = norm(cp-p_ist); %Abstand Carrot-Point zum Fahrzeug
    err = abs(1-dist/lad) %Normierung des Fehlers auf LAD

time_out = oldtime + dt; %Neuer Zeitpunkt, auf dem sich CP befindet, wird prognostiziert
end

== matlab function ZSM_TeslaModelS_statKreisfahrt/Vehicle/Betriebsstrategie/Momentenverteilung_und_Schaltstrategie1/Radmomentenaufteilung (Effizienz)/Momentenrückführung und Motormomentberechnung/Getriebewirkungsgradberechnung Hinterachse/MATLAB Function1 ==
  data: M_out input; M_in output; M_max input
function M_in = fcn(M_out, M_max)
M_in = 3/680 *((sqrt(M_max) * sqrt(27*M_max + 27200*M_out))/sqrt(3) - 3 * M_max)

== matlab function ZSM_TeslaModelS_statKreisfahrt/Vehicle/Antriebsstrang und Radmomentenverteilung/Batterie/MATLAB Function3 ==
  data: u input; y output
function y = fcn(u)
%Zusammenfassung der Verluste der LE auf eine Vektorspalte -> für das
%Batteriemodell


y=reshape(u,[[],1,1]);



end

== matlab function ZSM_TeslaModelS_statKreisfahrt/Vehicle/Antriebsstrang und Radmomentenverteilung/MATLAB Function2 ==
  data: u input; RIX output
function RIX = fcn(u)
%RIX = 1 für Antrieb an mindestens einem Rad, sonst -1
s = (sign(u) == 1);
if all(s) == 0
    RIX = -1;
else
    RIX = 1;
end
end

== matlab function ZSM_TeslaModelS_statKreisfahrt/Vehicle/Antriebsstrang und Radmomentenverteilung/MATLAB Function3 ==
  data: u input; RIX output
function RIX = fcn(u)
%RIX = 1 für Antrieb an mindestens einem Rad, sonst -1
s = (sign(u) == 1);
if all(s) == 0
    RIX = -1;
else
    RIX = 1;
end
end

== matlab function ZSM_TeslaModelS_statKreisfahrt/Vehicle/Betriebsstrategie/Momentenverteilung_und_Schaltstrategie1/Limitierungen gesamt (mit MVS Limits)/Aktuatoren und Delta TV/TV Moment pro Achse ==
  data: L1 input; Delta_T_f output; L2 input; L3 input; L4 input; L5 input; a_f input; a_r input; Delta_T_r output
function [Delta_T_f, Delta_T_r]  = fcn(L1, L2, L3, L4, L5, a_f, a_r)

%% Initialisierung
Delta_T_f=0;
Delta_T_r=0;

%% Zuweisung der maximalen TV Momente anhand der Antriebsstrangtopologie
if a_f == 3
    Delta_T_f=L5;
elseif a_f == 4
    Delta_T_f=L1;
elseif a_f == 5
    Delta_T_f=L2;
end

if a_r == 3
    Delta_T_r=L5;
elseif a_r == 4
    Delta_T_r=L1;
elseif a_r == 5
    Delta_T_r=L2;
end

%% Nomenklatur der Aktuatoren a_r und a_f
    % 1 = nur Elektromaschinen an der Achse
    % 2 = Offenes Differential an der Achse
    % 3 = Limited Slip Differential an der Achse
    % 4 = Elektrisches Überlagerungsgetriebe an der Achse
    % 5 = Mechanisches Überlagerungsgetriebe an der Achse

== matlab function ZSM_TeslaModelS_statKreisfahrt/Vehicle/Antriebsstrang und Radmomentenverteilung/MATLAB Function4 ==
  data: u input; RIX output
function RIX = fcn(u)
%RIX = 1 für Antrieb an mindestens einem Rad, sonst -1
s = (sign(u) == 1);
if all(s) == 0
    RIX = -1;
else
    RIX = 1;
end
end

== matlab function ZSM_TeslaModelS_statKreisfahrt/Vehicle/Antriebsstrang und Radmomentenverteilung/MATLAB Function5 ==
  data: u input; RIX output
function RIX = fcn(u)
%RIX = 1 für Antrieb an mindestens einem Rad, sonst -1
s = (sign(u) == 1);
if all(s) == 0
    RIX = -1;
else
    RIX = 1;
end
end

== matlab function ZSM_TeslaModelS_statKreisfahrt/Vehicle/Betriebsstrategie/Momentenverteilung_und_Schaltstrategie1/Limitierungen gesamt (mit MVS Limits)/Aktuatoren und Delta TV/Zuweisung Aktuatoren ==
  data: A1 input; A2 input; A3 input; A4 input; A5 input; a_f output; a_r output; A6 input; A7 input; A8 input; A9 input; A10 input
function [a_f, a_r]  = fcn(A1, A2, A3, A4, A5, A6, A7, A8, A9, A10)

%% Initialisierung
a_f=1;
a_r=1;

%% Zuweisung der Aktuatoren
% vorne
if A1 == 1
    a_f = 2;
elseif A2 == 1
    a_f = 3;
elseif A3 == 1
    a_f = 5;
elseif A4 == 1
    a_f = 4;
elseif A5 == 1
    a_f = 1;
end

% hinten
if A6 == 1
    a_r = 2;
elseif A7 == 1
    a_r = 3;
elseif A8 == 1
    a_r = 5;
elseif A9 == 1
    a_r = 4;
elseif A10 == 1
    a_r = 1;
end

%% Nomenklatur der Aktuatoren a_r und a_f
    % 1 = nur Elektromaschinen an der Achse
    % 2 = Offenes Differential an der Achse
    % 3 = Limited Slip Differential an der Achse
    % 4 = Elektrisches Überlagerungsgetriebe an der Achse
    % 5 = Mechanisches Überlagerungsgetriebe an der Achse

== matlab function ZSM_TeslaModelS_statKreisfahrt/Vehicle/Antriebsstrang und Radmomentenverteilung/MATLAB Function ==
  data: u input; RIX output
function RIX = fcn(u)
%RIX = 1 für Antrieb an mindestens einem Rad, sonst -1
s = (sign(u) == 1);
if all(s) == 0
    RIX = -1;
else
    RIX = 1;
end
end

== matlab function ZSM_TeslaModelS_statKreisfahrt/Vehicle/Antriebsstrang und Radmomentenverteilung/MATLAB Function1 ==
  data: u input; RIX output
function RIX = fcn(u)
%RIX = 1 für Antrieb an mindestens einem Rad, sonst -1
s = (sign(u) == 1);
if all(s) == 0
    RIX = -1;
else
    RIX = 1;
end
end

== matlab function ZSM_TeslaModelS_statKreisfahrt/Vehicle/Betriebsstrategie/Momentenverteilung_und_Schaltstrategie1/Limitierungen gesamt (mit MVS Limits)/Limits Zusammenführung ==
  data: FxlimRF input; FxlimLF input; FxlimRR input; Fx_LF_ub output; Fx_LF_lb output; Fx_RF_ub output; Fx_RF_lb output; Fx_LR_ub output; Fx_LR_lb output; Fx_RR_ub output; Fx_RR_lb output; FxlimLR input; M_RF_ub input; M_RF_lb input; M_LF_ub input; M_LF_lb input; M_RR_ub input; M_RR_lb input; M_LR_ub input; M_LR_lb input; M_F_lb input; M_F_ub input; M_R_lb input; M_R_ub input; DELTA_T_f input; DELTA_T_r input; a_f input; a_r input; r input
function [Fx_LF_ub, Fx_LF_lb, Fx_RF_ub, Fx_RF_lb, Fx_LR_ub, Fx_LR_lb, Fx_RR_ub, Fx_RR_lb] = fcn(FxlimRF, FxlimLF, FxlimRR, FxlimLR, M_RF_ub, M_RF_lb, M_LF_ub, M_LF_lb, M_RR_ub, M_RR_lb, M_LR_ub, M_LR_lb, M_F_lb, M_F_ub, M_R_lb, M_R_ub,DELTA_T_f, DELTA_T_r,a_f, a_r, r)

% Reifenverhalten beim Antreiben und Bremsen gleich
Fx_LF_ub = FxlimLF;
Fx_RF_ub = FxlimRF;
Fx_LF_lb = (-1*FxlimLF);
Fx_RF_lb = (-1*FxlimRF);

Fx_LR_ub = FxlimLR;
Fx_RR_ub = FxlimRR;
Fx_LR_lb = (-1*FxlimLR);
Fx_RR_lb = (-1*FxlimRR);

% Notwendig, da die Rekuperationskennfelder aus dem Pesche Tool positive
% Momente ausgeben
M_RF_lb=(-1)*M_RF_lb;
M_LF_lb=(-1)*M_LF_lb;
M_RR_lb=(-1)*M_RR_lb;
M_LR_lb=(-1)*M_LR_lb;
M_F_lb=(-1)*M_F_lb;
M_R_lb=(-1)*M_R_lb;
    
%% Nomenklatur der Aktuatoren a_r und a_f
    % 1 = nur Elektromaschinen an der Achse
    % 2 = Offenes Differential an der Achse
    % 3 = Limited Slip Differential an der Achse
    % 4 = Elektrisches Überlagerungsgetriebe an der Achse
    % 5 = Mechanisches Überlagerungsgetriebe an der Achse
 
    
%% Nur Elektromotoren: Limit ist Minimum/Maximum aus Reifenlimit und Limit der EM
if a_f == 1
    Fx_LF_ub = min(FxlimLF,(M_LF_ub/r));
    Fx_RF_ub = min(FxlimRF,(M_RF_ub/r));
    Fx_LF_lb = max((-1*FxlimLF),(M_LF_lb/r));
    Fx_RF_lb = max((-1*FxlimRF),(M_RF_lb/r));
end

if a_r == 1
    Fx_LR_ub = min(FxlimLR,(M_LR_ub/r));
    Fx_RR_ub = min(FxlimRR,(M_RR_ub/r));
    Fx_LR_lb = max((-1*FxlimLR),(M_LR_lb/r));
    Fx_RR_lb = max((-1*FxlimRR),(M_RR_lb/r));
end

%% Offenes Differential: Limit ist Minimum/Maximum aus Reifenlimit und genau der Hälfte des max. Moments der achszentralen EM
if a_f == 2
    Fx_LF_ub = min(FxlimLF,(0.5*M_F_ub/r));
    Fx_RF_ub = min(FxlimRF,(0.5*M_F_ub/r));
    Fx_LF_lb = max((-1*FxlimLF),(0.5*M_F_lb/r));
    Fx_RF_lb = max((-1*FxlimRF),(0.5*M_F_lb/r));
end

if a_r == 2
    Fx_LR_ub = min(FxlimLR,(0.5*M_R_ub/r));
    Fx_RR_ub = min(FxlimRR,(0.5*M_R_ub/r));
    Fx_LR_lb = max((-1*FxlimLR),(0.5*M_R_lb/r));
    Fx_RR_lb = max((-1*FxlimRR),(0.5*M_R_lb/r));
end

%% Limited Slip Differential %% Elektrisches Überlagerungsgetriebe %% Mechanisches Überlagerungsgetriebe:
if a_f >= 3 
    Fx_LF_ub = min(FxlimLF,(0.5*M_F_ub/r + 0.5*DELTA_T_f/r));
    Fx_RF_ub = min(FxlimRF,(0.5*M_F_ub/r + 0.5*DELTA_T_f/r));
    Fx_LF_lb = max((-1*FxlimLF),(0.5*M_F_lb/r - 0.5*DELTA_T_f/r));
    Fx_RF_lb = max((-1*FxlimRF),(0.5*M_F_lb/r - 0.5*DELTA_T_f/r));
end

if a_r >= 3
    Fx_LR_ub = min(FxlimLR,(0.5*M_R_ub/r + 0.5*DELTA_T_r/r));
    Fx_RR_ub = min(FxlimRR,(0.5*M_R_ub/r + 0.5*DELTA_T_r/r));
    Fx_LR_lb = max((-1*FxlimLR),(0.5*M_R_lb/r - 0.5*DELTA_T_r/r));
    Fx_RR_lb = max((-1*FxlimRR),(0.5*M_R_lb/r - 0.5*DELTA_T_r/r));
end


%% kein Antrieb an der achse
if a_f >= 4
    Fx_LF_ub = min(FxlimLF,(0.5*M_F_ub/r + 0.5*DELTA_T_f/r));
    Fx_RF_ub = min(FxlimRF,(0.5*M_F_ub/r + 0.5*DELTA_T_f/r));
    Fx_LF_lb = max((-1*FxlimLF),(0.5*M_F_lb/r - 0.5*DELTA_T_f/r));
    Fx_RF_lb = max((-1*FxlimRF),(0.5*M_F_lb/r - 0.5*DELTA_T_f/r));
end

if a_r >= 4
    Fx_LR_ub = min(FxlimLR,(0.5*M_R_ub/r + 0.5*DELTA_T_r/r));
    Fx_RR_ub = min(FxlimRR,(0.5*M_R_ub/r + 0.5*DELTA_T_r/r));
    Fx_LR_lb = max((-1*FxlimLR),(0.5*M_R_lb/r - 0.5*DELTA_T_r/r));
    Fx_RR_lb = max((-1*FxlimRR),(0.5*M_R_lb/r - 0.5*DELTA_T_r/r));
end

%% Torque Splitter
if a_f == 5
    Fx_LF_ub = min(FxlimLF,(M_F_ub/r));
    Fx_RF_ub = min(FxlimRF,(M_F_ub/r));
    Fx_LF_lb = max((-1*FxlimLF),(M_F_lb/r - DELTA_T_f/r));
    Fx_RF_lb = max((-1*FxlimRF),(M_F_lb/r - DELTA_T_f/r));
end

if a_r == 5
    Fx_LR_ub = min(FxlimLR,(M_R_ub/r));
    Fx_RR_ub = min(FxlimRR,(M_R_ub/r));
    Fx_LR_lb = max((-1*FxlimLR),(M_R_lb/r - DELTA_T_r/r));
    Fx_RR_lb = max((-1*FxlimRR),(M_R_lb/r - DELTA_T_r/r));
end

== matlab function ZSM_TeslaModelS_statKreisfahrt/Vehicle/Betriebsstrategie/Momentenverteilung_und_Schaltstrategie1/Radmomentenaufteilung (Effizienz)/Torque shift damper/Optimierung_eine_achs/Optimierung ==
  data: P_achs input; P_opt output; ind output; M_target input; VA input; HA input
function [P_opt, ind]= fcn(P_achs, M_target, VA, HA)

[n_gears, leng] = size(P_achs);

if HA == 1
    if M_target>0
        [P_opt, ind] = min(P_achs(:,1));
    else
        [P_opt, ind] = max(P_achs(:,1));
    end
else
    if M_target>0
        [P_opt, ind] = min(P_achs(:,leng));
    else
        [P_opt, ind] = max(P_achs(:,leng));
    end
    ind = ind+100*n_gears
end

end

== matlab function ZSM_TeslaModelS_statKreisfahrt/Vehicle/Betriebsstrategie/Momentenverteilung_und_Schaltstrategie1/Radmomentenaufteilung (Standardfahrmanöver)/Limits berücksichtigen ==
  data: Fx_RF output; Fx_LF output; Fx_RR output; Fx_LF_ub input; Fx_LF_lb input; Fx_RF_ub input; Fx_RF_lb input; Fx_LR_ub input; Fx_LR_lb input; Fx_RR_ub input; Fx_RR_lb input; a_f input; a_r input; Fx_LR output; X_FL input; X_FR input; X_RL input; X_RR input
function [Fx_RF, Fx_LF, Fx_RR, Fx_LR] = fcn(Fx_LF_ub, Fx_LF_lb, Fx_RF_ub, Fx_RF_lb, Fx_LR_ub, Fx_LR_lb, Fx_RR_ub, Fx_RR_lb,a_f, a_r, X_FL, X_FR, X_RL, X_RR)

%% Initialisierung
Fx_RF = X_FR;
Fx_LF = X_FL;
Fx_RR = X_RR;
Fx_LR = X_RL;
    
%% Nomenklatur der Aktuatoren a_r und a_f
    % 1 = nur Elektromaschinen an der Achse
    % 2 = Offenes Differential an der Achse
    % 3 = Limited Slip Differential an der Achse
    % 4 = Elektrisches Überlagerungsgetriebe an der Achse
    % 5 = Mechanisches Überlagerungsgetriebe an der Achse
 
%% Algorithmus

    F_f= Fx_RF+Fx_LF;
    F_r= Fx_RR+Fx_LR;
  
  % Nur Elektromotoren:
  % Es werden radindividuell die Grenzen eingehalten. Die Differenzkräfte
  % werden zur späteren Verwendung gespeichert.
if a_f ==1
    if Fx_LF > Fx_LF_ub
        dFx_LF = Fx_LF-Fx_LF_ub;
        Fx_LF = Fx_LF_ub;
    end
    if Fx_RF > Fx_RF_ub
        dFx_RF = Fx_RF-Fx_RF_ub;
        Fx_RF = Fx_RF_ub;
    end
    if Fx_LF < Fx_LF_lb
        dFx_LF = Fx_LF-Fx_LF_lb;
        Fx_LF = Fx_LF_lb;
    end
    if Fx_RF < Fx_RF_lb
        dFx_RF = Fx_RF-Fx_RF_lb;
        Fx_RF = Fx_RF_lb;
    end
end

if a_r ==1
    if Fx_LR > Fx_LR_ub
        dFx_LR = Fx_LR-Fx_LR_ub;
        Fx_LR = Fx_LR_ub;
    end
    if Fx_RR > Fx_RR_ub
        dFx_RR = Fx_RR-Fx_RR_ub;
        Fx_RR = Fx_RR_ub;
    end
    if Fx_LR < Fx_LR_lb
        dFx_LR = Fx_LR-Fx_LR_lb;
        Fx_LR = Fx_LR_lb;
    end
    if Fx_RR < Fx_RR_lb
        dFx_RR = Fx_RR-Fx_RR_lb;
        Fx_RR = Fx_RR_lb;
    end
end

  % Offenes Differential:
  % ALSO keine TV Funktion der Achse.
  % Jedes Rad erhält die Hälfte der Gesamtachskraft.
  % Anschließend wird diese Kraft auf das Minimum der einzelnen Limits
  % gedeckelt.

  %Berücksichtigung bereits in Lagrange-Block
  
if a_f ==2
    Fx_LF = F_f/2;
    Fx_RF = F_f/2;
    if Fx_LF > Fx_LF_ub || Fx_RF > Fx_RF_ub
        Fx_LF = min(Fx_LF_ub,Fx_RF_ub);
        Fx_RF = Fx_LF;
    end
    if Fx_LF < Fx_LF_lb || Fx_RF < Fx_RF_lb
        Fx_LF = max(Fx_LF_lb,Fx_RF_lb);
        Fx_RF = Fx_LF;
    end
end

if a_r ==2
    Fx_LR = F_r/2;
    Fx_RR = F_r/2;
    if Fx_LR > Fx_LR_ub || Fx_RR > Fx_RR_ub
        Fx_LR = min(Fx_LR_ub,Fx_RR_ub);
        Fx_RR = Fx_LR;
    end
    if Fx_LR < Fx_LR_lb || Fx_RR < Fx_RR_lb
        Fx_LR = max(Fx_LR_lb,Fx_RR_lb);
        Fx_RR = Fx_LR;
    end
end
    
%% Limited Slip Differential %% Elektrisches Überlagerungsgetriebe %% Mechanisches Überlagerungsgetriebe
if a_f >=3
    if Fx_LF > Fx_LF_ub
        dFx_LF = Fx_LF-Fx_LF_ub;
        Fx_LF = Fx_LF_ub;
    end
    if Fx_RF > Fx_RF_ub
        dFx_RF = Fx_RF-Fx_RF_ub;
        Fx_RF = Fx_RF_ub;
    end
    if Fx_LF < Fx_LF_lb
        dFx_LF = Fx_LF-Fx_LF_lb;
        Fx_LF = Fx_LF_lb;
    end
    if Fx_RF < Fx_RF_lb
        dFx_RF = Fx_RF-Fx_RF_lb;
        Fx_RF = Fx_RF_lb;
    end
end

if a_r >=3
    if Fx_LR > Fx_LR_ub
        dFx_LR = Fx_LR-Fx_LR_ub;
        Fx_LR = Fx_LR_ub;
    end
    if Fx_RR > Fx_RR_ub
        dFx_RR = Fx_RR-Fx_RR_ub;
        Fx_RR = Fx_RR_ub;
    end
    if Fx_LR < Fx_LR_lb
        dFx_LR = Fx_LR-Fx_LR_lb;
        Fx_LR = Fx_LR_lb;
    end
    if Fx_RR < Fx_RR_lb
        dFx_RR = Fx_RR-Fx_RR_lb;
        Fx_RR = Fx_RR_lb;
    end
end
    
%% Korrektur des TV Moments %% Korrektur des Gesamtmoments

== matlab function ZSM_TeslaModelS_statKreisfahrt/Vehicle/Betriebsstrategie/Momentenverteilung_und_Schaltstrategie1/Radmomentenaufteilung (Effizienz)/Torque shift damper/Optimierung_damped_AWD/Minimierung ==
  data: P_achs input; P_opt output; ind output; count output; difference input; max_oscillation_sec input; M_target input; change input; ind_prev input; count_prev input
function [P_opt, ind, count]= fcn(P_achs, difference, max_oscillation_sec, M_target, change, ind_prev, count_prev)

[leng, x] = size(P_achs);
if M_target>0
    [P_opt, ind] = min(P_achs(:));

    if (P_opt < (1-difference)*P_achs(ind_prev) && count_prev > (leng*2000/max_oscillation_sec)) || change == -1 || isnan(P_achs(ind_prev)) == 1
        count = 0
    else
        ind = ind_prev;
        P_opt = P_achs(ind_prev);
        count = count_prev+1;
    end

else
    [P_opt, ind] = max(P_achs(:));
    
    if (P_opt > (1+difference)*P_achs(ind_prev) && count_prev > (leng*2000/max_oscillation_sec)) || change == -1 || isnan(P_achs(ind_prev)) == 1
        count = 0
    else
        ind = ind_prev;
        P_opt = P_achs(ind_prev);
        count = count_prev+1;
    end
end

end

== matlab function ZSM_TeslaModelS_statKreisfahrt/Vehicle/Betriebsstrategie/Momentenverteilung_und_Schaltstrategie1/Radmomentenaufteilung (Standardfahrmanöver)/Optimierung mit Lagrange Multiplikator Methode ==
  data: a_f input; a_r input; X_req input; Z_FL input; Z_FR input; Z_RL input; Z_RR input; Mz input; tF input; tR input; lf input; lr input; delta input; X_FL output; X_FR output; X_RL output; X_RR output; X_FL1 input; X_FR1 input; X_RL1 input; X_RR1 input
function [X_FL, X_FR, X_RL, X_RR] = fcn(a_f, a_r, X_req, Z_FL, Z_FR, Z_RL, Z_RR, Mz, tF, tR, lf, lr, delta, X_FL1, X_FR1, X_RL1, X_RR1)

%% Auswahl der Antriebsstrantopologie
a=1;
b=1;

if a_f ==2
    a=0;
end
if a_r ==2
    b=0;
end

if a_f ==2 && a_r==2
    a=1;
    b=1;
end

% TV vorne und hinten möglich a=1 und b=1
% TV nur vorne möglich a=1
% TV nur hinten möglich b=1
% kein TV möglich a=1 und b=1 und anschließend gleichmäßig aufteilen

%% Matrix für die Randbedingungen ( Gesamtmoment und TV Moment)
% B0 = [cos(delta) cos(delta) 1 1; a*((-tF/2)*cos(delta)+lf*sin(delta)) a*((tF/2)*cos(delta)+lf*sin(delta)) b*(-tR/2) b*(tR/2)];
% Die Berücksichtigung der Lenkwinkel für die Formel des Gesamtmoments und des Giermomenmts ist exakt, wird
% aber hier erstmal auskommentiert, da ein instabiler Fahrerregler
% vorliegt. Sobald der Fahrerregler komplett stabil ist, kann die obere
% Matrix für B0 verwendet werden.
B0 = [1 1 1 1; a*(-tF/2) a*(tF/2) b*(-tR/2) b*(tR/2)];
y0 = [X_req; Mz];

%% Algorithmus
    %% Initialbedingungen
i=0;    
B=B0;
y=y0;
     
    %% Verhindern abgehobener Räder
if Z_FL < 1
    Z_FL = 1;
    x_FL_max = 0;
end

if Z_FR < 1
    Z_FR = 1;
    x_FR_max = 0;
end

if Z_RL < 1
    Z_RL = 1;
    x_RL_max = 0;
end

if Z_RR < 1
    Z_RR = 1;
    x_RR_max = 0;
end

%% Matrizen für die Mimimierung
W1 = [1/Z_FL 0 0 0; 0 1/Z_FR 0 0; 0 0 1/Z_RL 0; 0 0 0 1/Z_RR];
W2 = 0.01 * eye(4);
%Wquad = W1^2 + W2^2;
Wquad = W1 + W2^2;
X_alt = [X_FL1; X_FR1; X_RL1; X_RR1];

%% Minimierungsargument
% min ||W1*x||^2 + ||W2*(x-x0)||^2
%   ||W1*x||^2 + ||W2*(x-x0)||^2 = xt*W1^2*x + (x-x0)t*W2^2*(x-x0)
%   = xt*(W1^2+W2^2)*x - 2*x*W2^2*x0 + x0*W2^2*x0
%   = xt*W^2*x - 2*x*W2^2*x0 + Konstante
%   mit W^2 = W1^2 + W2^2

%% Berechnung von Xij
G = (Wquad^(-1))*(B')*(B*(Wquad^(-1))*(B'))^(-1);
X = G*y + (eye(4)-G*B)*(Wquad^(-1))*(W2^2)*X_alt;


%% Ausgabewerte berechnen
X_FL = X(1);
X_FR = X(2);
X_RL = X(3);
X_RR = X(4);

%% Limits berücksichtigen
if a==0
    X_F = X_FL + X_FR;
    X_FL = X_F/2;
    X_FR = X_F/2;
end

if b==0
    X_R = X_RL + X_RR;
    X_RL = X_R/2;
    X_RR = X_R/2;
end

if a_f ==2 && a_r==2
    X_F = X_FL + X_FR;
    X_FL = X_F/2;
    X_FR = X_F/2;
    X_R = X_RL + X_RR;
    X_RL = X_R/2;
    X_RR = X_R/2;
end

== matlab function ZSM_TeslaModelS_statKreisfahrt/Vehicle/Betriebsstrategie/Momentenverteilung_und_Schaltstrategie1/Radmomentenaufteilung (Standardfahrmanöver)/Schaltstrategie/Getriebe- wirkungs- grade ==
  data: eta_LF output; eta_RF output; eta_LR output; eta_RR output; eta_F output; eta_R output; idx_LF input; idx_RF input; idx_LR input; idx_RR input; idx_F input; idx_R input; ETA_F input; ETA_R input
function [eta_LF, eta_RF, eta_LR, eta_RR, eta_F, eta_R] = fcn(idx_LF, idx_RF, idx_LR, idx_RR, idx_F, idx_R, ETA_F, ETA_R)

eta_LF=ETA_F(idx_LF);
eta_RF=ETA_F(idx_RF);
eta_LR=ETA_R(idx_LR);
eta_RR=ETA_R(idx_RR);
eta_F=ETA_F(idx_F);
eta_R=ETA_R(idx_R);

% Der Wirkungsgrad des Getriebes im eingelegten Gang wird weitergegeben.
% Frederik benötigt diesen im Antriebsstrangmodell.

== matlab function ZSM_TeslaModelS_statKreisfahrt/Vehicle/Betriebsstrategie/Momentenverteilung_und_Schaltstrategie1/Radmomentenaufteilung (Standardfahrmanöver)/Schaltstrategie/Radmoment zu Motormoment ==
  data: i_LF input; i_RF input; i_LR input; i_RR input; i_F input; i_R input; M_LF input; m_LF output; M_RF input; M_LR input; M_RR input; m_RF output; m_LR output; m_RR output; m_F output; m_R output
function [m_LF, m_RF, m_LR, m_RR, m_F, m_R] = fcn(i_LF, i_RF, i_LR, i_RR, i_F, i_R, M_LF, M_RF, M_LR, M_RR)

%% Motormoment Achszentraler Aufbau
m_F=(M_LF+M_RF)/i_F;
m_R=(M_LR+M_RR)/i_R;

%% Motormoment Radindividueller Aufbau
m_LF=M_LF/i_LF;
m_RF=M_RF/i_RF;
m_LR=M_LR/i_LR;
m_RR=M_RR/i_RR;
